simulink model "ImpulseGen"  (Simulink 8.9)
settings: Solver=ode45  StartTime=0.0  StopTime=120.0  MaxStep=.05  RelTol=1e-3  AbsTol=1e-6
undefined symbols (not defined in the file or in its folder): sfunyst
settings Model: SuppressorTable=22 serialization::archive 11 0 6 0 0 0 11 0  Creator=vise  LastModifiedBy=dangd  ExtModeTrigMode=oneshot  ExtModeArmWhenConnect=off  ExtModeAutoUpdateStatusClock=off
settings DataIOCC: LimitDataPoints=off
settings OptimizationCC: BooleanDataType=off  ExpressionDepthLimit=2147483647  InitFltsAndDblsToZero=on
settings DebuggingCC: SaveWithParameterizedLinksMsg=none  SignalResolutionControl=TryResolveAllWithWarning  MultiTaskDSMMsg=warning  MultiTaskCondExecSysMsg=none
settings HardwareCC: TargetUnknown=on
settings RTWCC: TemplateMakefile=grt_unix.tmf
settings GRTTargetCC: GeneratePreprocessorConditionals=Use local settings

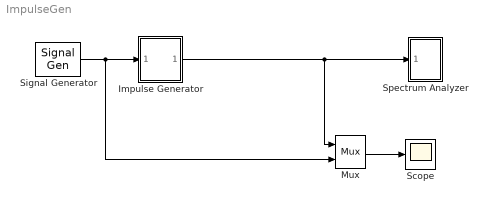
== system ImpulseGen ==
  Impulse Generator : Subsystem  mask(D-T interpolator){T=1, MaskParam2=0.3}
      mask prompts: T "Input sampling period:"; MaskParam2 "Pulse width:"
      mask init:
      | L=round(T/MaskParam2);
      mask Display: plot(-10,-10,110,110,[0,50,50,60,60,100],[0,0,80,80,0,0])
  Mux : Mux  Inputs=2
  Scope : Scope
  Signal Generator : SignalGenerator  Amplitude=1.000000  Frequency=0.8
  Spectrum Analyzer : Subsystem  LoadFcn=sfunyst([],[],[],'LoadBlock')  mask(Spectrum analyzer.){N=2048, T_s=0.05, plot_period=10}
      mask prompts: N "Number of sample points:"; T_s "Sampling period (sec):"; plot_period "Plotting Period (sec):"
      settings: CopyFcn=sfunyst([],[],[],'CopyBlock')  DeleteFcn=sfunyst([],[],[],'DeleteBlock')
      mask Help: EE438 Lab utility; See Prof. Bouman.
      mask Display: plot(0,0,100,100,[14,91,91,14,14],[86,86,40,40,86],[85,82,80,79,75,67,63,60,57,53,41,36,33,27,24],[49,50,53,50,49,51,54,66,54,50,50,52,81,51,49])
  wires:
  Mux/1 -> Scope/1
  Signal Generator/1 -> Mux/2, Impulse Generator/1(in_1)
  Impulse Generator/1(out_1) -> Mux/1, Spectrum Analyzer/1(input signal)

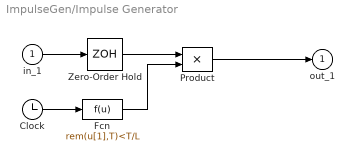
== system ImpulseGen/Impulse Generator ==
  in_1 : Inport
  Clock : Clock
  Fcn : Fcn  Expr=rem(u[1],T)<T/L
  Product : Product  SaturateOnIntegerOverflow=on  RndMeth=Zero  InputSameDT=on  OutDataTypeStr=Inherit: Same as first input
  Zero-Order Hold : ZeroOrderHold  SampleTime=T
  out_1 : Outport  InitialOutput=0
  wires:
  in_1/1 -> Zero-Order Hold/1
  Zero-Order Hold/1 -> Product/1
  Fcn/1 -> Product/2
  Product/1 -> out_1/1
  Clock/1 -> Fcn/1

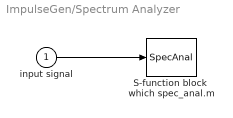
== system ImpulseGen/Spectrum Analyzer ==
  input signal : Inport
  S-function block  which spec_anal.m : S-Function  FunctionName=SpecAnal  Parameters=N,T_s,plot_period  SFunctionDeploymentMode=off  EnableBusSupport=off
  wires:
  input signal/1 -> S-function block  which spec_anal.m/1
